simulink model "wind_model"  (R2020a)
settings: Solver=FixedStepAuto  StartTime=0.0  StopTime=10.0  RelTol=1e-3
PreLoadFcn:
  | load("interfaces.mat");
libraries: simulink x2, simulink_extras x1
settings Model: Creator=thomas.evang  LastModifiedBy=thomas.evang
settings SFSimCC: CustomCodeUndefinedFunction=UseInterfaceOnly
settings RTWCC: Description=FMU based on GRT (Functional Mock-up Unit)  SystemTargetFile=grtfmi.tlc  GenerateMakefile=off  TemplateMakefile=none  RetainRTWFile=on
settings STFCustomTargetCC: TargetLangStandard=C99 (ISO)  CombineOutputUpdateFcns=on  MultiInstanceERTCode=on  CodeInterfacePackaging=Reusable function  GenerateAllocFcn=on  SystemTargetFile=grtfmi.tlc
settings GRTTargetCC: ParMdlRefBuildCompliant=off  CompOptLevelCompliant=off  ConcurrentExecutionCompliant=off  MatFileLogging=off  MultiInstanceERTCode=on  CodeInterfacePackaging=Reusable function  CPPClassGenCompliant=off  GenerateAllocFcn=on  UseToolchainInfoCompliant=off

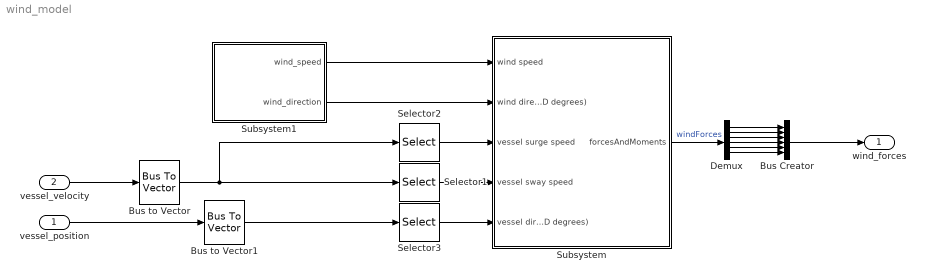
== system wind_model ==
  vessel_position : Inport  OutDataTypeStr=Bus: position_6dof
  vessel_velocity : Inport  Port=2  OutDataTypeStr=Bus: velocity_6dof
  Bus Creator : BusCreator  Inputs=6  OutDataTypeStr=Bus: force_6dof
      settings: InheritFromInputs=off
  Bus to Vector : BusToVector
  Bus to Vector1 : BusToVector
  Demux : Demux  Outputs=6
  Selector1 : Selector  InputPortWidth=6  IndexOptions=Index vector (dialog)  Indices=2  OutputSizes=1
  Selector2 : Selector  InputPortWidth=6  IndexOptions=Index vector (dialog)  Indices=1  OutputSizes=1
  Selector3 : Selector  InputPortWidth=6  IndexOptions=Index vector (dialog)  Indices=6  OutputSizes=1
  Subsystem : Subsystem
  Subsystem1 : Subsystem  mask{uMean=10, thetaMeanDegrees=0}
      mask prompts: uMean "Mean Wind Speed"; thetaMeanDegrees "Mean Wind Direction"
  wind_forces : Outport  OutDataTypeStr=Bus: force_6dof  VectorParamsAs1DForOutWhenUnconnected=off
  wires:
  Bus Creator/1 -> wind_forces/1
  Demux/2 -> Bus Creator/2
  vessel_velocity/1 -> Bus to Vector/1
  Demux/1 -> Bus Creator/1
  Selector2/1 -> Subsystem/3(vessel surge speed)
  Selector3/1 -> Subsystem/5(vessel direction (NED degrees))
  Subsystem1/1(wind_speed) -> Subsystem/1(wind speed)
  Bus to Vector/1 -> Selector1/1, Selector2/1
  Demux/4 -> Bus Creator/4
  Selector1/1 -> Subsystem/4(vessel sway speed)
  Demux/3 -> Bus Creator/3
  Subsystem1/2(wind_direction) -> Subsystem/2(wind direction (NED degrees))
  Demux/5 -> Bus Creator/5
  Subsystem/1(forcesAndMoments) -> Demux/1  "windForces"
  Demux/6 -> Bus Creator/6
  vessel_position/1 -> Bus to Vector1/1
  Bus to Vector1/1 -> Selector3/1

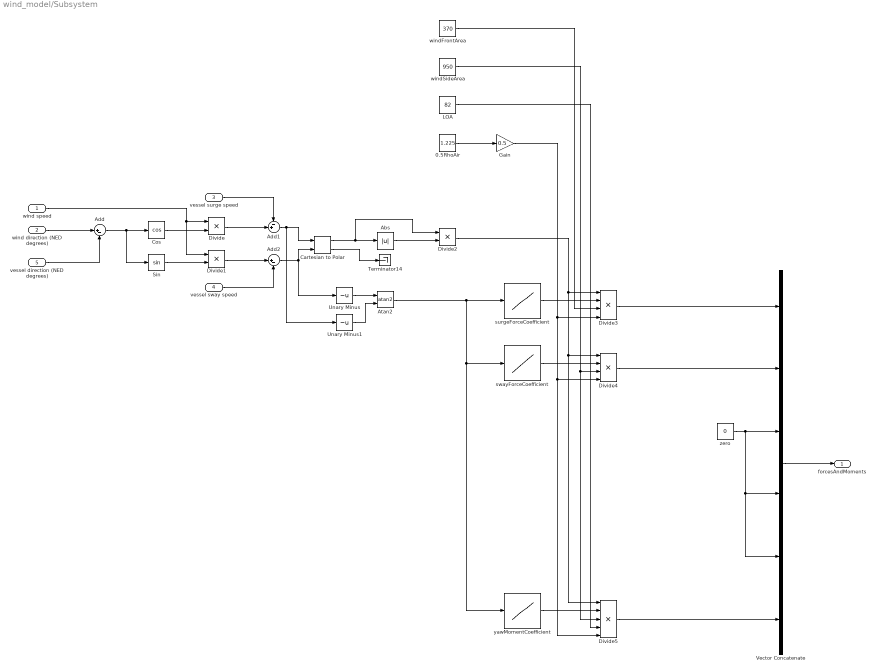
== system wind_model/Subsystem ==
  wind speed : Inport
  wind direction (NED degrees) : Inport  Port=2
  vessel surge speed : Inport  Port=3
  vessel sway speed : Inport  Port=4
  vessel direction (NED degrees) : Inport  Port=5
  0.5RhoAir : Constant  Value=1.225
  Abs : Abs
  Add : Sum  Inputs=|+-
  Add1 : Sum  Inputs=-+|
  Add2 : Sum  Inputs=|+-
  Atan2 : Trigonometry  Operator=atan2
  Cartesian to Polar : simulink_extras/Transformations/Cartesian to Polar
  Cos : Trigonometry  Operator=cos
  Divide : Product
  Divide1 : Product
  Divide2 : Product
  Divide3 : Product  Inputs=4
  Divide4 : Product  Inputs=4
  Divide5 : Product  Inputs=5
  Gain : Gain  Gain=0.5
  LOA : Constant  Value=82
  Sin : Trigonometry
  Terminator14 : Terminator
  Unary Minus : UnaryMinus
  Unary Minus1 : UnaryMinus
  Vector Concatenate : Concatenate  NumInputs=6
  surgeForceCoefficient : Lookup_n-D  NumberOfTableDimensions=1  BreakpointsForDimension1=[0:10:360]  Table=[-0.55 -0.56 -0.50 -0.49 -0.42 -0.34 -0.24 -0.17 -0.11 -0.09 -0.05 0.08 0.39 0.59 0.72 0.80 0.76 0.81 0.80 0.81 0.76 0.80 0.72 0.59 0.39 0.08 -0.05 -0.09 -0.11 -0.17 -0.24 -0.34 -0.42 -0.49 -0.50 -0.56 -0.55]  InternalRulePriority=Speed  RndMeth=Simplest  InputSameDT=on
  swayForceCoefficient : Lookup_n-D  NumberOfTableDimensions=1  BreakpointsForDimension1=[0:10:360]  Table=|  InternalRulePriority=Speed  RndMeth=Simplest  InputSameDT=on
      | [0.0	-0.21	-0.40	-0.60	-0.76	-0.84	-0.95	-0.97	-0.96	-0.92	-0.91	-0.90	-0.86	-0.76	-0.66	-0.51	-0.31	-0.09	0	0.09	0.31	0.51	0.66	0.76	0.86	0.9	0.91	0.92	0.96	0.97	0.95	0.84	0.76	0.6	0.4	0.21	0
      | ]
  windFrontArea : Constant  Value=370
  windSideArea : Constant  Value=950
  yawMomentCoefficient : Lookup_n-D  NumberOfTableDimensions=1  BreakpointsForDimension1=[0:10:360]  Table=|  InternalRulePriority=Speed  RndMeth=Simplest  InputSameDT=on
      | [0.0	-0.060	-0.111	-0.150	-0.160	-0.161	-0.172	-0.162	-0.131	-0.108	-0.071	-0.047	-0.032	-0.008	0.002	0.005	0.007	0.016	0.0	-0.016	-0.007	-0.005	-0.002	0.008	0.032	0.047	0.071	0.108	0.131	0.162	0.172	0.161	0.16	0.15	0.111	0.06	0
      | ]
  zero : Constant  Value=0
  forcesAndMoments : Outport  VectorParamsAs1DForOutWhenUnconnected=off
  wires:
  wind speed/1 -> Divide1/1, Divide/1
  Divide1/1 -> Add2/1
  Gain/1 -> Divide5/5, Divide4/4, Divide3/4
  Add/1 -> Sin/1, Cos/1
  Sin/1 -> Divide1/2
  Divide/1 -> Add1/2
  vessel direction (NED degrees)/1 -> Add/2
  zero/1 -> Vector Concatenate/4, Vector Concatenate/5, Vector Concatenate/3
  wind direction (NED degrees)/1 -> Add/1
  Divide4/1 -> Vector Concatenate/2
  LOA/1 -> Divide5/4
  yawMomentCoefficient/1 -> Divide5/2
  vessel surge speed/1 -> Add1/1
  Divide2/1 -> Divide3/1, Divide4/1, Divide5/1
  Add2/1 -> Unary Minus/1, Cartesian to Polar/2
  windFrontArea/1 -> Divide3/3
  Divide3/1 -> Vector Concatenate/1
  Cartesian to Polar/1 -> Divide2/1, Abs/1
  Divide5/1 -> Vector Concatenate/6
  Add1/1 -> Unary Minus1/1, Cartesian to Polar/1
  Vector Concatenate/1 -> forcesAndMoments/1
  Cartesian to Polar/2 -> Terminator14/1
  surgeForceCoefficient/1 -> Divide3/2
  Atan2/1 -> yawMomentCoefficient/1, swayForceCoefficient/1, surgeForceCoefficient/1
  windSideArea/1 -> Divide5/3, Divide4/3
  Unary Minus/1 -> Atan2/1
  Abs/1 -> Divide2/2
  vessel sway speed/1 -> Add2/2
  Cos/1 -> Divide/2
  0.5RhoAir/1 -> Gain/1
  swayForceCoefficient/1 -> Divide4/2
  Unary Minus1/1 -> Atan2/2

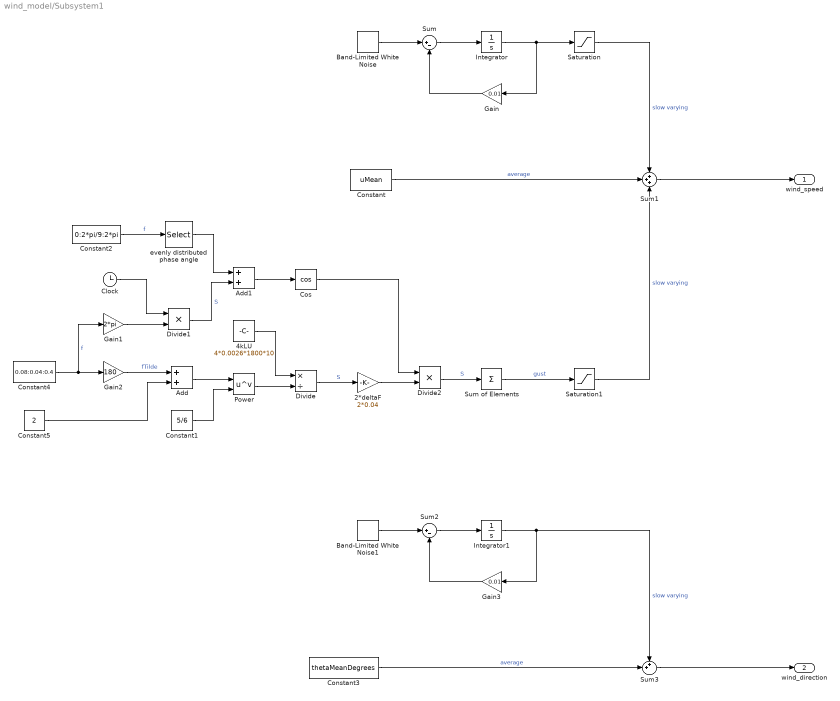
== system wind_model/Subsystem1 ==
  2*deltaF : Gain  Gain=2*0.04
  4kLU : Constant  Value=4*0.0026*1800*10
  Add : Sum
  Add1 : Sum
  Band-Limited White Noise : simulink/Sources/Band-Limited White Noise  Cov=[0.1]  Ts=0.1  seed=[23341]
  Band-Limited White Noise1 : simulink/Sources/Band-Limited White Noise  Cov=[0.1]  Ts=0.1  seed=[23342]
  Clock : Clock
  Constant : Constant  Value=uMean
  Constant1 : Constant  Value=5/6
  Constant2 : Constant  Value=0:2*pi/9:2*pi
  Constant3 : Constant  Value=thetaMeanDegrees
  Constant4 : Constant  Value=0.08:0.04:0.4
  Constant5 : Constant  Value=2
  Cos : Trigonometry  Operator=cos
  Divide : Product  Inputs=*/
  Divide1 : Product
  Divide2 : Product
  Gain : Gain  Gain=0.01
  Gain1 : Gain  Gain=2*pi
  Gain2 : Gain  Gain=180
  Gain3 : Gain  Gain=0.01
  Integrator : Integrator
  Integrator1 : Integrator
  Power : Math  Operator=pow  SignedPower=on  SaturateOnIntegerOverflow=on
  Saturation : Saturate  UpperLimit=uMean/5  LowerLimit=-uMean/5
  Saturation1 : Saturate  UpperLimit=uMean/2  LowerLimit=-uMean/2
  Sum : Sum  Inputs=|+-
  Sum of Elements : Sum  Inputs=+
  Sum1 : Sum  Inputs=+++
  Sum2 : Sum  Inputs=|+-
  Sum3 : Sum  Inputs=++|
  evenly distributed phase angle : Selector  InputPortWidth=10  IndexOptions=Index vector (dialog)  Indices=[1:9]  OutputSizes=1
  wind_speed : Outport  VectorParamsAs1DForOutWhenUnconnected=off
  wind_direction : Outport  Port=2  VectorParamsAs1DForOutWhenUnconnected=off
  wires:
  Band-Limited White Noise1/1 -> Sum2/1
  Constant3/1 -> Sum3/2  "average"
  Gain3/1 -> Sum2/2
  Saturation1/1 -> Sum1/3  "slow varying"
  Gain1/1 -> Divide1/2
  evenly distributed phase angle/1 -> Add1/1
  Sum of Elements/1 -> Saturation1/1  "gust"
  Constant/1 -> Sum1/2  "average"
  Clock/1 -> Divide1/1
  Sum3/1 -> wind_direction/1
  Sum/1 -> Integrator/1
  Sum1/1 -> wind_speed/1
  Integrator1/1 -> Sum3/1, Gain3/1  "slow varying"
  Sum2/1 -> Integrator1/1
  Constant2/1 -> evenly distributed phase angle/1  "f"
  Divide2/1 -> Sum of Elements/1  "S"
  Constant4/1 -> Gain1/1, Gain2/1  "f"
  Add1/1 -> Cos/1
  Integrator/1 -> Gain/1, Saturation/1
  4kLU/1 -> Divide/1
  Divide1/1 -> Add1/2  "S"
  Cos/1 -> Divide2/1
  Gain/1 -> Sum/2
  Divide/1 -> 2*deltaF/1  "S"
  Constant1/1 -> Power/2
  2*deltaF/1 -> Divide2/2
  Constant5/1 -> Add/2
  Add/1 -> Power/1
  Saturation/1 -> Sum1/1  "slow varying"
  Band-Limited White Noise/1 -> Sum/1
  Power/1 -> Divide/2
  Gain2/1 -> Add/1  "fTilde"
